simulink model "compare_setup_nonlinear"  (R2021b)
settings: Solver=ode45  StartTime=0.0  StopTime=10  RelTol=1e-3  EnableMultiTasking=on
values from neighbouring files (symbols this model uses):
  A = double(A)    [step4_0_linearize_operating_point.m]    (also in step4_linearized_system.mat = [0 -1.79155728996 0 111.114105003 0 1 -687.855245355 0 1440.)
  adingain = [adin_gain 1 1 1 1 1]    [hwinit.m]
  adinoffs = [-adin_offs 0 0 0 0 0]    [hwinit.m]
  B = double(B)    [step4_0_linearize_operating_point.m]    (also in step4_linearized_system.mat = [0 0 0 0 2553.84140127])
  C = [1 0 0 0 0 ... (first row only)    [step4_0_linearize_operating_point.m]    (also in step4_linearized_system.mat = [1  0  0  0  0; 0  0  1  0  0])
  D = zeros(2,1)    [step4_0_linearize_operating_point.m]    (also in step4_linearized_system.mat = [0 0])
  daoutgain = 1*[-6]    [hwinit.m]
  daoutoffs = [0.00]    [hwinit.m]
  g1 = (m_1 * c_1_0 + m_2 * l_1) * g    [compare_ourmodel_with_others.m]    (also in step4_0_linearize_operating_point.m = (m1 * c1 + m2 * l1) * g; step6_1_controller_feedback.m = (m1 * c1 + m2 * l1) * g)
  g2 = m_2 * c_2_0 * g    [compare_ourmodel_with_others.m]    (also in step4_0_linearize_operating_point.m = m2 * c2 * g; step6_1_controller_feedback.m = m2 * c2 * g)
  h = 0.001    [hwinit.m]    (also in init_fugi.m = fugiboard('Open', 'pendulum1'); rotpentest.m = fugiboard('Open', 'pendulum1'))
  P1 = m_1 * c_1_0 * c_1_0 + m_2 * l_1 * l_1 + I_1_0    [compare_ourmodel_with_others.m]    (also in step4_0_linearize_operating_point.m = m1 * c1 * c1 + m2 * l1 * l1 + I1; step6_1_controller_feedback.m = m1 * c1 * c1 + m2 * l1 * l1 + I1)
  P2 = m_2 * c_2_0 * c_2_0 + I_2_0    [compare_ourmodel_with_others.m]    (also in step4_0_linearize_operating_point.m = m2 * c2 * c2 + I2; step6_1_controller_feedback.m = m2 * c2 * c2 + I2)
  P3 = m_2 * l_1 * c_2_0    [compare_ourmodel_with_others.m]    (also in step4_0_linearize_operating_point.m = m2 * l1 * c2; step6_1_controller_feedback.m = m2 * l1 * c2)
  params = [9.81, 0.1, 0.1, 0.125, 0.0487, -0.0286, 0.0624, 0.0169, 6.81e-5, 6.9742, 2.89e-05, 46.1069, 0.0308]    [compare_ourmodel_with_others.m]    (also in costfun.m = x; step2_whitebox_pend.m = x; step4_linearized_system.mat = [9.81 0.1 0.1 0.125 0.046955 -0.032 0.04609 0.0088 9.8e-05 6)
  theta_1_0 = pi    (= 3.14159265359)    [hwinit.m]    (also in step4_0_linearize_operating_point.m = 0; step6_1_controller_feedback.m = 0)
  theta_2_0 = 0    [hwinit.m]    (also in step4_0_linearize_operating_point.m; step6_1_controller_feedback.m)
  x_op = [theta_1_0; 0; theta_2_0; 0; 0]    [step4_0_linearize_operating_point.m]    (also in step4_linearized_system.mat = [0 0 0 0 0])
settings Model: Creator=rbabuska  LastModifiedBy=lyitingli
settings SolverCC: AlgebraicLoopSolver=TrustRegion
settings DataIOCC: LimitDataPoints=on  SaveFormat=Array  ReturnWorkspaceOutputs=off  SignalLoggingName=sigsOut
settings OptimizationCC: BooleanDataType=off  ExpressionDepthLimit=2147483647  InitFltsAndDblsToZero=on  LifeSpan=inf
settings DebuggingCC: SaveWithParameterizedLinksMsg=none  SignalResolutionControl=TryResolveAllWithWarning  MultiTaskDSMMsg=warning  MultiTaskCondExecSysMsg=none  AllowSymbolicDim=off  StateNameClashWarn=warning  SFUnexpectedBacktrackingDiag=warning  SFNoUnconditionalDefaultTransitionDiag=warning  SFExecutionAtInitializationDiag=none  SFMachineParentedDataDiag=warning  ArithmeticOperatorsInVariantConditions=warning
settings HardwareCC: ProdBitPerPointer=32  ProdBitPerSizeT=32  ProdBitPerPtrDiffT=32  ProdLargestAtomicFloat=None  ProdIntDivRoundTo=Undefined  ProdEndianess=Unspecified  ProdWordSize=32  ProdHWDeviceType=32-bit Generic  TargetUnknown=on
settings ModelReferenceCC: PropagateSignalLabelsOutOfModel=off
settings SFSimCC: SimUseLocalCustomCode=off  CustomCodeUndefinedFunction=UseInterfaceOnly
settings RTWCC: RTWUseLocalCustomCode=off
settings CodeAppCC: StateflowObjectComments=on
settings GRTTargetCC: TargetFcnLib=ansi_tfl_tmw.mat  TargetLangStandard=C89/C90 (ANSI)  CombineOutputUpdateFcns=off  GRTInterface=on
settings ConfigComp: CovMetricSettings=dw  CovSaveCumulativeToWorkspaceVar=on  CovSaveSingleToWorkspaceVar=on  CovExternalEMLEnable=off

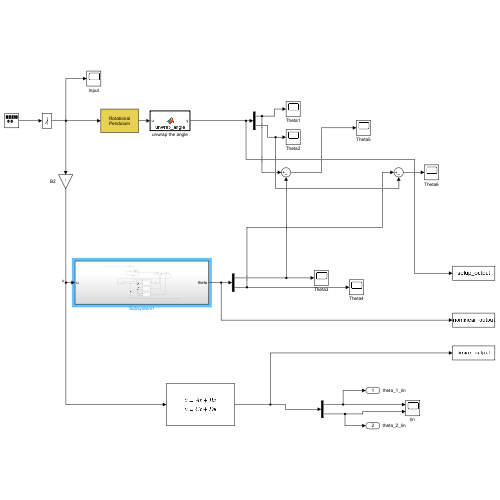
[thumbnail: Simulink's stored preview of the top-level diagram]
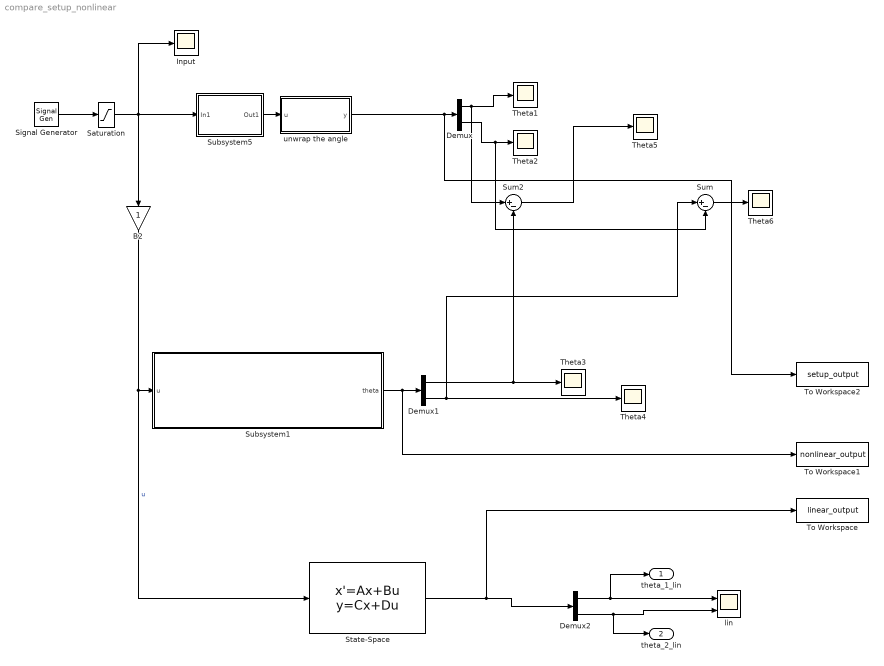
== system compare_setup_nonlinear ==
  B2 : Gain
  Demux : Demux  Outputs=2
  Demux1 : Demux  Outputs=2
  Demux2 : Demux  Outputs=2
  Input : Scope
  Saturation : Saturate  UpperLimit=1  LowerLimit=-1
  Signal Generator : SignalGenerator  Amplitude=0.5  Frequency=0.5
  State-Space : StateSpace  A=A  B=B  C=C  D=D  InitialCondition=x_op-x_op
  Subsystem1 : Subsystem
  Subsystem5 : Subsystem
      mask Display: disp('Rotational\nPendulum')
  Sum : Sum  Inputs=|+-
  Sum2 : Sum  Inputs=|+-
  Theta{1..6} (6 alike) : Scope
  To Workspace : ToWorkspace  VariableName=linear_output  SampleTime=0.001
  To Workspace1 : ToWorkspace  VariableName=nonlinear_output  SampleTime=0.001
  To Workspace2 : ToWorkspace  VariableName=setup_output  SampleTime=0.001
  lin : Scope  NumInputPorts=2
  unwrap the angle : MATLAB Function  TreatAsAtomicUnit=on
  theta_1_lin : Outport
  theta_2_lin : Outport  Port=2
  wires:
  Demux/1 -> Theta1/1, Sum2/1
  Subsystem5/1(Out1) -> unwrap the angle/1(u)
  Signal Generator/1 -> Saturation/1
  Saturation/1 -> B2/1, Subsystem5/1(In1), Input/1
  Demux1/1 -> Theta3/1, Sum2/2
  Demux1/2 -> Theta4/1, Sum/1
  Demux/2 -> Sum/2, Theta2/1
  Sum2/1 -> Theta5/1
  Sum/1 -> Theta6/1
  Subsystem1/1(theta) -> To Workspace1/1, Demux1/1
  B2/1 -> State-Space/1, Subsystem1/1(u)  "u"
  Demux2/2 -> lin/2, theta_2_lin/1
  State-Space/1 -> To Workspace/1, Demux2/1
  Demux2/1 -> theta_1_lin/1, lin/1
  unwrap the angle/1(y) -> To Workspace2/1, Demux/1

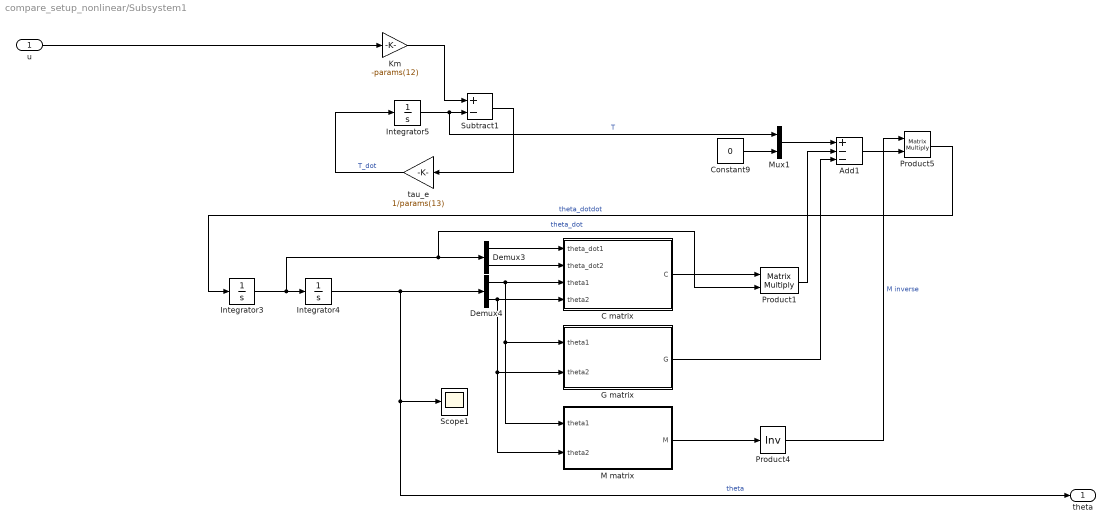
== system compare_setup_nonlinear/Subsystem1 ==
  u : Inport
  Add1 : Sum  Inputs=+--
  C matrix : MATLAB Function  TreatAsAtomicUnit=on
  Constant9 : Constant  Value=0
  Demux3 : Demux  Outputs=2
  Demux4 : Demux  Outputs=2
  G matrix : MATLAB Function  TreatAsAtomicUnit=on
  Integrator3 : Integrator
  Integrator4 : Integrator  InitialCondition=[theta_1_0 theta_2_0]
  Integrator5 : Integrator
  Km : Gain  Gain=-params(12)
  M matrix : MATLAB Function  TreatAsAtomicUnit=on
  Mux1 : Mux  Inputs=2
  Product1 : Product  Inputs=**  Multiplication=Matrix(*)
  Product4 : Product  Inputs=/  Multiplication=Matrix(*)
  Product5 : Product  Inputs=**  Multiplication=Matrix(*)
  Scope1 : Scope
  Subtract1 : Sum  Inputs=+-
  tau_e : Gain  Gain=1/params(13)
  theta : Outport
  wires:
  Demux4/1 -> M matrix/1(theta1), G matrix/1(theta1), C matrix/3(theta1)
  tau_e/1 -> Integrator5/1  "T_dot"
  Constant9/1 -> Mux1/2
  Demux3/1 -> C matrix/1(theta_dot1)
  Add1/1 -> Product5/2
  Subtract1/1 -> tau_e/1
  G matrix/1(G) -> Add1/3
  Integrator3/1 -> Product1/2, Demux3/1, Integrator4/1  "theta_dot"
  C matrix/1(C) -> Product1/1
  Mux1/1 -> Add1/1
  Integrator5/1 -> Mux1/1, Subtract1/2  "T"
  u/1 -> Km/1
  Product5/1 -> Integrator3/1  "theta_dotdot"
  Demux3/2 -> C matrix/2(theta_dot2)
  Integrator4/1 -> Demux4/1, theta/1, Scope1/1  "theta"
  M matrix/1(M) -> Product4/1
  Demux4/2 -> M matrix/2(theta2), G matrix/2(theta2), C matrix/4(theta2)
  Product4/1 -> Product5/1  "M inverse"
  Product1/1 -> Add1/2
  Km/1 -> Subtract1/1

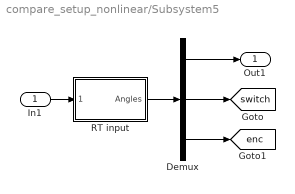
== system compare_setup_nonlinear/Subsystem5 ==
  In1 : Inport
  Demux : Demux  Outputs=[2 4 1]
  RT input : Subsystem  mask{Ts=h, channels=[6 7]}
      mask prompts: Ts "Sample time [s]:"; channels "Channels to read (e.g., [6 7])"
      mask init:
      | hwinit;
      | 
      | % initialize FPGA
      | fugihandle = fugiboard('Open', 'Pendulum1');
      | fugihandle.WatchdogTimeout = 0.5;
      | fugiboard('SetParams', fugihandle);
      | fugiboard('Write', fugihandle, 0, 0, 0, 0);  % dummy write to sync interface board
      | fugiboard('Write', fugihandle, 5, 1, 0, 0);  % reset position, activate relay
      | data = fugiboard('Read', fugihandle);        % get version info from FPGA
      | % model = bitshift(data(1), -5); 
      | % version = bitand(data(1), 31);
      | % disp(sprintf('FPGA setup %d, version %d', model, version)); % for the B&P it should say 1 1, or else there is a problem
      | fugiboard('Write', fugihandle, 0, 1, 0, 0);  % end reset
      | pause(0.1);                         % give relay some time to respond
      mask Display: disp('Rotational\nPendulum')
  Out1 : Outport
  tag scope: enc=global, switch=global
  wires:
  RT input/1(Angles) -> Demux/1
  Demux/1 -> Out1/1
  Demux/2 -> [switch]
  Demux/3 -> [enc]
  In1/1 -> RT input/1(Motors)

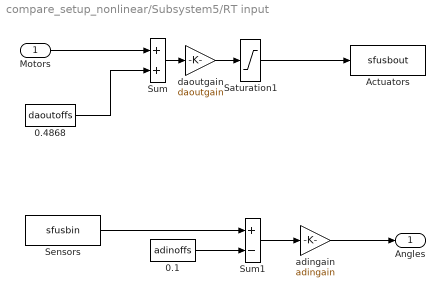
== system compare_setup_nonlinear/Subsystem5/RT input ==
  Motors : Inport
  0.1 : Constant  Value=adinoffs
  0.4868 : Constant  Value=daoutoffs
  Actuators : S-Function  FunctionName=sfusbout  Parameters=Ts, fugihandle  SFunctionDeploymentMode=off  EnableBusSupport=off
  Saturation1 : Saturate  UpperLimit=10  LowerLimit=-10
  Sensors : S-Function  FunctionName=sfusbin  Parameters=Ts, fugihandle, channels  SFunctionDeploymentMode=off  EnableBusSupport=off
  Sum : Sum  InputSameDT=on  SaturateOnIntegerOverflow=on  OutDataTypeStr=Inherit: Same as first input
  Sum1 : Sum  Inputs=+-  InputSameDT=on  SaturateOnIntegerOverflow=on  OutDataTypeStr=Inherit: Same as first input
  adingain : Gain  Gain=adingain  SaturateOnIntegerOverflow=on  OutDataTypeStr=Inherit: Same as input  ParamDataTypeStr=Inherit: Same as input
  daoutgain : Gain  Gain=daoutgain  SaturateOnIntegerOverflow=on  OutDataTypeStr=Inherit: Same as input  ParamDataTypeStr=Inherit: Same as input
  Angles : Outport
  wires:
  Sum/1 -> daoutgain/1
  0.4868/1 -> Sum/2
  Motors/1 -> Sum/1
  Sum1/1 -> adingain/1
  0.1/1 -> Sum1/2
  adingain/1 -> Angles/1
  Saturation1/1 -> Actuators/1
  daoutgain/1 -> Saturation1/1
  Sensors/1 -> Sum1/1

== matlab function compare_setup_nonlinear/unwrap the angle ==
  settings: updateMethod=DISCRETE  sampleTime=0.001
  data: u input size=2; y output size=2
function y = unwrap_angle(u)

y = unwrap(u);
y = u;

== matlab function compare_setup_nonlinear/Subsystem1/C matrix ==
  data: theta_dot1 input; theta_dot2 input; theta1 input; theta2 input; C output; params parameter; P3 parameter
function C = C(theta_dot1, theta_dot2, theta1, theta2, params, P3)
c00 = params(10) - P3 * theta_dot2 * sin(theta2);
c01 = -P3 * (theta_dot1 + theta_dot2) * sin(theta2);
c10 = P3 * theta_dot1 * sin(theta2);
c11 = params(11);

C = [c00 c01;
     c10 c11];

== matlab function compare_setup_nonlinear/Subsystem1/G matrix ==
  data: theta1 input; theta2 input; G output; g1 parameter; g2 parameter
function G = G(theta1, theta2, g1, g2)
G00 = -g1 * sin(theta1) - g2 * sin(theta1 + theta2);
G01 = -g2 * sin(theta1 + theta2);

G = [G00 G01];

== matlab function compare_setup_nonlinear/Subsystem1/M matrix ==
  data: theta1 input; theta2 input; M output; P1 parameter; P2 parameter; P3 parameter
function M = fcn(theta1, theta2, P1, P2, P3)
M00 = P1 + P2 + 2 * P3 * cos(theta2);
M01 = P2 + P3 * cos(theta2);
M10 = M01;
M11 = P2;

M = [M00 M01;
     M10 M11];
